simulink model "crossroad_cs"  (R2021a)
settings: Solver=ode5  StartTime=0.0  StopTime=50  FixedStep=1/1000  RelTol=1e-3
PreLoadFcn:
  | mbxruntime.callbacks.PreLoadFcn(bdroot);
PostLoadFcn:
  | mbxruntime.callbacks.PostLoadFcn(bdroot);
InitFcn:
  | mbxruntime.callbacks.InitFcn(bdroot);
StartFcn:
  | mbxruntime.callbacks.StartFcn(bdroot);
StopFcn:
  | mbxruntime.callbacks.StopFcn(bdroot);
model workspace: external: MAT-File .\crossroad_cs_hws.mat (data not in the file)
values from neighbouring files (symbols this model uses):
  c_factor = 43.75    [emplanner_init.m]
  cf = -175016    [emplanner_init.m]
  cr = -130634    [emplanner_init.m]
  KD_PID_distance = 0.0    (= 0)    [emplanner_init.m]
  KD_PID_speed = 0    [emplanner_init.m]
  KI_PID_distance = 0.0    (= 0)    [emplanner_init.m]
  KI_PID_speed = 0    [emplanner_init.m]
  KP_PID_distance = 0.5    [emplanner_init.m]
  KP_PID_speed = 1.8    [emplanner_init.m]
  la = 1.265    [emplanner_init.m]
  lb = 2.947-1.265    (= 1.682)    [emplanner_init.m]
  LQR_K1 = k(:,1)'    [emplanner_init.m]
  LQR_K2 = k(:,2)'    [emplanner_init.m]
  LQR_K3 = k(:,3)'    [emplanner_init.m]
  LQR_K4 = k(:,4)'    [emplanner_init.m]
  m = 2020    [emplanner_init.m]
  my_global_path_x = [0.4409 0.940746626271 1.44028225507 1.93950267328 2.43840536558 2.93698884522 3.43525224935 3.93319509352 4.43081712279 4.92811822143 5.42509835808 5.92175755256 ... (6001 elements, 6001x1)]    [my_global_path.mat]    (also in my_global_path_200.mat = [0.4409 0.940746626271 1.44028225507 1.93950267328 2.4384053)
  my_global_path_y = [58.2244 58.2243999975 58.2243999675 58.2243998683 58.224399668 58.2243993499 58.2243989099 58.2243983526 58.2243976886 58.2243969324 58.2243961011 58.2243952132 ... (6001 elements, 6001x1)]    [my_global_path.mat]    (also in my_global_path_200.mat = [58.2244 58.2243999975 58.2243999675 58.2243998683 58.224399)
  rack_displacement = [-39.14 , -37.2 , -35.29 , -33.43 , -31.6 , -29.81 , -28.06 , -26.34 , -24.66 ,      -23.01 , -21.38 , -19.79 , -18.23 , -16.69 , -15.18 , -13.7 , -12.23 , -10.8 , -9.38 , -7.98 ,     -6.61 , -5.25 , -3.91 , -2.59 , -1.29 , 0 , 1.27 , 2.54 , 3.78 , 5.02 , 6.24 , 7.46 , 8.66 ,      9.86 , 11.05 , 12.24 , 13.41 , 14.59 , 15.76 , 16.92 , 18.09 , 19.25 , 20.42 , 21.59 , 22.76 ,      23.93 , 25.11 , 26 ...(+26 chars)    [emplanner_init.m]
  right_wheel_ground = [-70 ,-67.2 , -64.4 , -61.6 , -58.8 , -56 , -53.2 , -50.4 , -47.6 , -44.8 , -42 ,      -39.2 , -36.4 , -33.6 , -30.8 , -28 , -25.2 , -22.4 , -19.6 , -16.8 , -14 , -11.2 , -8.4 , -5.6 ,      -2.8 , 0 , 2.8 , 5.6 , 8.4 , 11.2 , 14 , 16.8 , 19.6 , 22.4 , 25.2 , 28 , 30.8 , 33.6 , 36.4 ,      39.2 , 42 , 44.8 , 47.6 , 50.4 , 53.2 , 56 , 58.8 , 61.6 , 64.4 , 67.2 , 70 ]    [emplanner_init.m]
  vx_break_point = zeros(1,5000)    [emplanner_init.m]
undefined symbols (not defined in the file or in its folder): aubr, DiscIntNeverNeededParam, tablebr, vubr
libraries: PreScanSimulinkLibrary x11, Solver_SF x1
(part 4 of 8)

== system crossroad_cs/Box_3/Dynamics_Empty/MuxState ==
  note: mode: Dynamics
  note: mode: Positioning
  note: mode: Dynamics
      | VelVEHICLE
      | wrt VEH
  note: AnglesVEHICLE
      | wrtGLOB
  note: For state mode 'Dynamic' positions
      | are not taken into account, as they
      | are computed by integrating velocity.
      | Click annotation for Help.
  x [m] : Inport  SampleTime=TimeStep
  y [m] : Inport  Port=2  SampleTime=TimeStep
  z [m] : Inport  Port=3  SampleTime=TimeStep
  dx [m/s] : Inport  Port=4  SampleTime=TimeStep
  dy [m/s] : Inport  Port=5  SampleTime=TimeStep
  dz [m/s] : Inport  Port=6  SampleTime=TimeStep
  R [rad] : Inport  Port=7  SampleTime=TimeStep
  P [rad] : Inport  Port=8  SampleTime=TimeStep
  Y [rad] : Inport  Port=9  SampleTime=TimeStep
  Constant : Constant  DisableCoverage=on  Value=positioningmode
  Discrete-Time Integrator : DiscreteIntegrator  SampleTime=TimeStep  ICPrevOutput=DiscIntNeverNeededParam  ICPrevScaledInput=DiscIntNeverNeededParam
  Ground : Ground
  Ground1 : Ground
  Mux1 : Mux  Inputs=[3 3]
  Mux2 : Mux  Inputs=3
  Mux3 : Mux  Inputs=3
  Mux4 : Mux  Inputs=3
  Mux5 : Mux  Inputs=[3 3]
  Mux6 : Mux  Inputs=[6 3]
  Switch : Switch  Threshold=0.5
  Transformation_BODY2GLOBAL : PreScanSimulinkLibrary/Simple_Vehicle_Dynamics/Chassis/MuxDynState/Transformation_BODY2GLOBAL  SystemSampleTime=-1  VariantActivationTime=update diagram  Latency=0  AutoFrameSizeCalculation=off
  mux3 : Mux  Inputs=3
  state : Outport
  wires:
  Constant/1 -> Switch/2
  Mux6/1 -> state/1
  Mux4/1 -> Mux1/1
  Mux5/1 -> Switch/3
  Mux1/1 -> Switch/1
  Switch/1 -> Mux6/1  "PosVeh wrt  GLOB"
  P [rad]/1 -> Mux3/2
  R [rad]/1 -> Mux3/1
  dz [m/s]/1 -> Mux2/3
  dy [m/s]/1 -> Mux2/2
  dx [m/s]/1 -> Mux2/1
  z [m]/1 -> Mux4/3
  y [m]/1 -> Mux4/2
  x [m]/1 -> Mux4/1
  Ground1/1 -> mux3/2  "pitch"
  Y [rad]/1 -> mux3/3, Mux3/3  "yaw"
  Mux3/1 -> Mux6/2
  Transformation_BODY2GLOBAL/1 -> Discrete-Time Integrator/1, Mux5/2  "VelVEH wrt  GLOB"
  mux3/1 -> Transformation_BODY2GLOBAL/2
  Ground/1 -> mux3/1  "roll"
  Mux2/1 -> Mux1/2, Transformation_BODY2GLOBAL/1
  Discrete-Time Integrator/1 -> Mux5/1  "PosVEH wrt  GLOB"

== system crossroad_cs/Box_3/Dynamics_Empty/STATE_Box_3 ==
  State : Inport  SampleTime=TimeStep
  Bus Creator : BusCreator  Inputs=15  OutDataTypeStr=Bus: PRESCAN_STATEACTUATORDATA  NonVirtualBus=on
  Constant : Constant  Value=0
  Demux : Demux  Outputs=15
  Mux : Mux  Inputs=3
  Mux1 : Mux  Inputs=3
  Mux2 : Mux  Inputs=3
  iniBODYAngles wrtVEH [rad] : Constant  Value=Roll0  SampleTime=TimeStep
  iniBODYAngles wrtVEH [rad]1 : Constant  Value=Pitch0  SampleTime=TimeStep
  iniVEHAngles wrtGLOB [rad] : Constant  Value=Yaw0  SampleTime=TimeStep
  iniVEHposition wrtGLOB [m] : Constant  Value=x0  SampleTime=TimeStep
  iniVEHposition wrtGLOB [m]1 : Constant  Value=y0  SampleTime=TimeStep
  iniVEHposition wrtGLOB [m]2 : Constant  Value=z0  SampleTime=TimeStep
  state2FullState : PreScanSimulinkLibrary/state2FullState  SystemSampleTime=-1  VariantActivationTime=update diagram  Latency=0  AutoFrameSizeCalculation=off
  StateBus : Outport  OutDataTypeStr=Bus: PRESCAN_STATEACTUATORDATA
  wires:
  Mux2/1 -> state2FullState/4
  iniVEHAngles wrtGLOB [rad]/1 -> Mux2/3
  Mux1/1 -> state2FullState/3
  Constant/1 -> Mux2/1, Mux2/2, Mux1/3
  iniBODYAngles wrtVEH [rad]1/1 -> Mux1/2
  iniBODYAngles wrtVEH [rad]/1 -> Mux1/1
  Mux/1 -> state2FullState/2
  iniVEHposition wrtGLOB [m]2/1 -> Mux/3
  iniVEHposition wrtGLOB [m]/1 -> Mux/1
  iniVEHposition wrtGLOB [m]1/1 -> Mux/2
  Demux/15 -> Bus Creator/15  "AngularVelocityYaw"
  Demux/14 -> Bus Creator/14  "AngularVelocityPitch"
  Demux/13 -> Bus Creator/13  "AngularVelocityRoll"
  Demux/12 -> Bus Creator/12  "OrientationYaw"
  Demux/11 -> Bus Creator/11  "OrientationPitch"
  Demux/10 -> Bus Creator/10  "OrientationRoll"
  Demux/9 -> Bus Creator/9  "AccelerationZ"
  Demux/8 -> Bus Creator/8  "AccelerationY"
  Demux/7 -> Bus Creator/7  "AccelerationX"
  Demux/6 -> Bus Creator/6  "VelocityZ"
  Demux/5 -> Bus Creator/5  "VelocityY"
  Demux/4 -> Bus Creator/4  "VelocityX"
  Demux/3 -> Bus Creator/3  "PositionZ"
  Demux/2 -> Bus Creator/2  "PositionY"
  Demux/1 -> Bus Creator/1  "PositionX"
  state2FullState/1 -> Demux/1
  State/1 -> state2FullState/1
  Bus Creator/1 -> StateBus/1

== system crossroad_cs/Box_3/SELF_Demux/compas converter ==
  rotz [rad] : Inport
  cart2compas : Subsystem
  rad2deg : Gain  Gain=180/pi
  heading [deg] : Outport
  wires:
  rad2deg/1 -> cart2compas/1(Angle [deg])
  rotz [rad]/1 -> rad2deg/1
  cart2compas/1(heading [deg]) -> heading [deg]/1

== system crossroad_cs/Box_4/Dynamics_Empty/MuxState ==
  note: mode: Dynamics
  note: mode: Positioning
  note: mode: Dynamics
      | VelVEHICLE
      | wrt VEH
  note: AnglesVEHICLE
      | wrtGLOB
  note: For state mode 'Dynamic' positions
      | are not taken into account, as they
      | are computed by integrating velocity.
      | Click annotation for Help.
  x [m] : Inport  SampleTime=TimeStep
  y [m] : Inport  Port=2  SampleTime=TimeStep
  z [m] : Inport  Port=3  SampleTime=TimeStep
  dx [m/s] : Inport  Port=4  SampleTime=TimeStep
  dy [m/s] : Inport  Port=5  SampleTime=TimeStep
  dz [m/s] : Inport  Port=6  SampleTime=TimeStep
  R [rad] : Inport  Port=7  SampleTime=TimeStep
  P [rad] : Inport  Port=8  SampleTime=TimeStep
  Y [rad] : Inport  Port=9  SampleTime=TimeStep
  Constant : Constant  DisableCoverage=on  Value=positioningmode
  Discrete-Time Integrator : DiscreteIntegrator  SampleTime=TimeStep  ICPrevOutput=DiscIntNeverNeededParam  ICPrevScaledInput=DiscIntNeverNeededParam
  Ground : Ground
  Ground1 : Ground
  Mux1 : Mux  Inputs=[3 3]
  Mux2 : Mux  Inputs=3
  Mux3 : Mux  Inputs=3
  Mux4 : Mux  Inputs=3
  Mux5 : Mux  Inputs=[3 3]
  Mux6 : Mux  Inputs=[6 3]
  Switch : Switch  Threshold=0.5
  Transformation_BODY2GLOBAL : PreScanSimulinkLibrary/Simple_Vehicle_Dynamics/Chassis/MuxDynState/Transformation_BODY2GLOBAL  SystemSampleTime=-1  VariantActivationTime=update diagram  Latency=0  AutoFrameSizeCalculation=off
  mux3 : Mux  Inputs=3
  state : Outport
  wires:
  Constant/1 -> Switch/2
  Mux6/1 -> state/1
  Mux4/1 -> Mux1/1
  Mux5/1 -> Switch/3
  Mux1/1 -> Switch/1
  Switch/1 -> Mux6/1  "PosVeh wrt  GLOB"
  P [rad]/1 -> Mux3/2
  R [rad]/1 -> Mux3/1
  dz [m/s]/1 -> Mux2/3
  dy [m/s]/1 -> Mux2/2
  dx [m/s]/1 -> Mux2/1
  z [m]/1 -> Mux4/3
  y [m]/1 -> Mux4/2
  x [m]/1 -> Mux4/1
  Ground1/1 -> mux3/2  "pitch"
  Y [rad]/1 -> mux3/3, Mux3/3  "yaw"
  Mux3/1 -> Mux6/2
  Transformation_BODY2GLOBAL/1 -> Discrete-Time Integrator/1, Mux5/2  "VelVEH wrt  GLOB"
  mux3/1 -> Transformation_BODY2GLOBAL/2
  Ground/1 -> mux3/1  "roll"
  Mux2/1 -> Mux1/2, Transformation_BODY2GLOBAL/1
  Discrete-Time Integrator/1 -> Mux5/1  "PosVEH wrt  GLOB"

== system crossroad_cs/Box_4/Dynamics_Empty/STATE_Box_4 ==
  State : Inport  SampleTime=TimeStep
  Bus Creator : BusCreator  Inputs=15  OutDataTypeStr=Bus: PRESCAN_STATEACTUATORDATA  NonVirtualBus=on
  Constant : Constant  Value=0
  Demux : Demux  Outputs=15
  Mux : Mux  Inputs=3
  Mux1 : Mux  Inputs=3
  Mux2 : Mux  Inputs=3
  iniBODYAngles wrtVEH [rad] : Constant  Value=Roll0  SampleTime=TimeStep
  iniBODYAngles wrtVEH [rad]1 : Constant  Value=Pitch0  SampleTime=TimeStep
  iniVEHAngles wrtGLOB [rad] : Constant  Value=Yaw0  SampleTime=TimeStep
  iniVEHposition wrtGLOB [m] : Constant  Value=x0  SampleTime=TimeStep
  iniVEHposition wrtGLOB [m]1 : Constant  Value=y0  SampleTime=TimeStep
  iniVEHposition wrtGLOB [m]2 : Constant  Value=z0  SampleTime=TimeStep
  state2FullState : PreScanSimulinkLibrary/state2FullState  SystemSampleTime=-1  VariantActivationTime=update diagram  Latency=0  AutoFrameSizeCalculation=off
  StateBus : Outport  OutDataTypeStr=Bus: PRESCAN_STATEACTUATORDATA
  wires:
  Mux2/1 -> state2FullState/4
  iniVEHAngles wrtGLOB [rad]/1 -> Mux2/3
  Mux1/1 -> state2FullState/3
  Constant/1 -> Mux2/1, Mux2/2, Mux1/3
  iniBODYAngles wrtVEH [rad]1/1 -> Mux1/2
  iniBODYAngles wrtVEH [rad]/1 -> Mux1/1
  Mux/1 -> state2FullState/2
  iniVEHposition wrtGLOB [m]2/1 -> Mux/3
  iniVEHposition wrtGLOB [m]/1 -> Mux/1
  iniVEHposition wrtGLOB [m]1/1 -> Mux/2
  Demux/15 -> Bus Creator/15  "AngularVelocityYaw"
  Demux/14 -> Bus Creator/14  "AngularVelocityPitch"
  Demux/13 -> Bus Creator/13  "AngularVelocityRoll"
  Demux/12 -> Bus Creator/12  "OrientationYaw"
  Demux/11 -> Bus Creator/11  "OrientationPitch"
  Demux/10 -> Bus Creator/10  "OrientationRoll"
  Demux/9 -> Bus Creator/9  "AccelerationZ"
  Demux/8 -> Bus Creator/8  "AccelerationY"
  Demux/7 -> Bus Creator/7  "AccelerationX"
  Demux/6 -> Bus Creator/6  "VelocityZ"
  Demux/5 -> Bus Creator/5  "VelocityY"
  Demux/4 -> Bus Creator/4  "VelocityX"
  Demux/3 -> Bus Creator/3  "PositionZ"
  Demux/2 -> Bus Creator/2  "PositionY"
  Demux/1 -> Bus Creator/1  "PositionX"
  state2FullState/1 -> Demux/1
  State/1 -> state2FullState/1
  Bus Creator/1 -> StateBus/1

== system crossroad_cs/Box_4/SELF_Demux/compas converter ==
  rotz [rad] : Inport
  cart2compas : Subsystem
  rad2deg : Gain  Gain=180/pi
  heading [deg] : Outport
  wires:
  rad2deg/1 -> cart2compas/1(Angle [deg])
  rotz [rad]/1 -> rad2deg/1
  cart2compas/1(heading [deg]) -> heading [deg]/1

== system crossroad_cs/Audi_A8_Sedan_1/Dynamics_UserSpecified/CarSim2PreScanSTATE/Transformation_SprungMassCarSim2PreScan ==
  In1 : Inport
  Demux : Demux  Outputs=3
  Ini z-position VEHICLE wrt GLOBAL axis system [m] : Constant  Value=z0
  Mux : Mux  Inputs=3
  Sum1 : Sum  Inputs=+-
  Out1 : Outport
  wires:
  Mux/1 -> Out1/1
  Ini z-position VEHICLE wrt GLOBAL axis system [m]/1 -> Sum1/2
  Demux/1 -> Mux/1
  Sum1/1 -> Mux/3
  Demux/3 -> Sum1/1
  Demux/2 -> Mux/2
  In1/1 -> Demux/1

== system crossroad_cs/Audi_A8_Sedan_1/SELF_Demux/compas converter/cart2compas ==
  Angle [deg] : Inport
  Constant : Constant  Value=90
  Constant1 : Constant  Value=360
  Gain : Gain  Gain=1/360
  Gain1 : Gain  Gain=360
  Gain2 : Gain  Gain=-1
  Rounding Function : Rounding
  Sum : Sum  Inputs=|-+
  Sum1 : Sum  Inputs=-+|
  Sum2 : Sum  Inputs=++|
  heading [deg] : Outport
  wires:
  Gain/1 -> Rounding Function/1
  Rounding Function/1 -> Gain1/1
  Gain1/1 -> Sum/1
  Angle [deg]/1 -> Sum1/2
  Sum/1 -> Gain2/1
  Sum1/1 -> Gain/1, Sum/2
  Constant/1 -> Sum1/1
  Gain2/1 -> Sum2/2
  Constant1/1 -> Sum2/1
  Sum2/1 -> heading [deg]/1

== system crossroad_cs/Audi_A8_Sedan_1/control module1/control main/chassic steering system ==
  LQR_final_angle : Inport
  Constant : Constant  Value=la
  Constant1 : Constant  Value=lb
  Constant17 : Constant  Value=c_factor
  Divide : Product  Inputs=*/
  Gain3 : Gain  Gain=180/pi
  Gain4 : Gain  Gain=360
  MATLAB Function : MATLAB Function  TreatAsAtomicUnit=on
  Saturation : Saturate  UpperLimit=70  LowerLimit=-70
  Saturation1 : Saturate  UpperLimit=1.2217  LowerLimit=-1.2217
  transfer right wheel angle to rack displancement : Lookup_n-D  NumberOfTableDimensions=1  BreakpointsForDimension1=right_wheel_ground  Table=rack_displacement  InternalRulePriority=Speed  RndMeth=Simplest  InputSameDT=on
  lat_steer_sw[deg] : Outport
  wires:
  transfer right wheel angle to rack displancement/1 -> Divide/1
  Constant17/1 -> Divide/2
  Gain4/1 -> lat_steer_sw[deg]/1
  Divide/1 -> Gain4/1
  Saturation/1 -> transfer right wheel angle to rack displancement/1
  Constant/1 -> MATLAB Function/2(la)
  Gain3/1 -> Saturation/1
  Constant1/1 -> MATLAB Function/3(lb)
  LQR_final_angle/1 -> Saturation1/1
  Saturation1/1 -> MATLAB Function/1(u)
  MATLAB Function/1(right_steer) -> Gain3/1

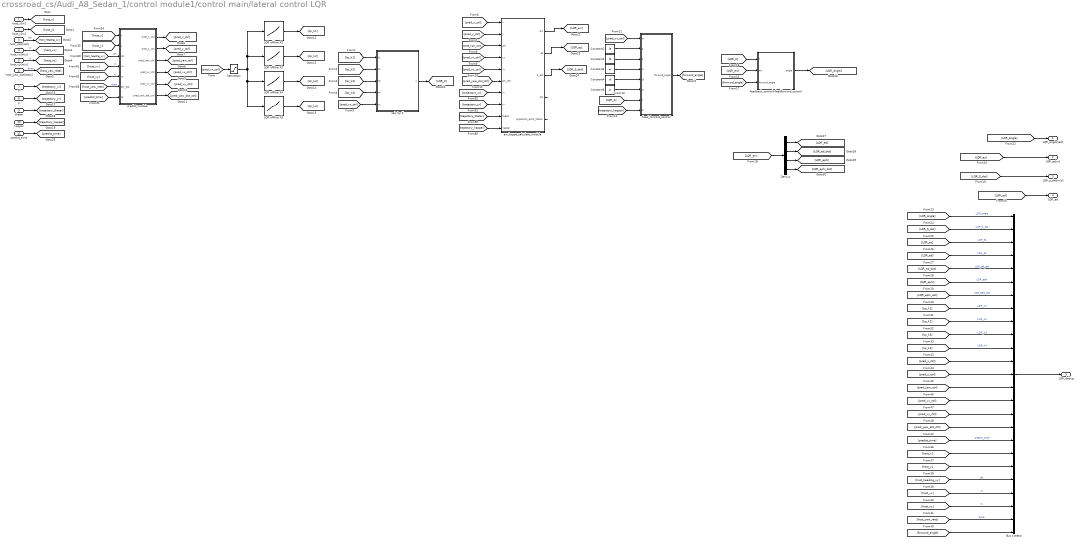
== system crossroad_cs/Audi_A8_Sedan_1/control module1/control main/lateral control LQR ==
  host_x[m] : Inport
  host_y[m] : Inport  Port=2
  host_yaw[rad] : Inport  Port=3
  host_vx[m/s] : Inport  Port=4
  host_vy[m/s] : Inport  Port=5
  host_yaw_dot[rad/s] : Inport  Port=6
  xr : Inport  Port=7
  yr : Inport  Port=8
  thetar : Inport  Port=9
  kappar : Inport  Port=10
  predict_time : Inport  Port=11
  Bus Creator : BusCreator  Inputs=25
  Constant1 : Constant  Value=la
  Constant2 : Constant  Value=lb
  Constant3 : Constant  Value=m
  Constant4 : Constant  Value=cf
  Constant5 : Constant  Value=cr
  Demux : Demux
  LQR offline K1 : Lookup_n-D  NumberOfTableDimensions=1  BreakpointsForDimension1=vx_break_point  Table=LQR_K1  InternalRulePriority=Speed  RndMeth=Simplest  InputSameDT=on
  LQR offline K2 : Lookup_n-D  NumberOfTableDimensions=1  BreakpointsForDimension1=vx_break_point  Table=LQR_K2  InternalRulePriority=Speed  RndMeth=Simplest  InputSameDT=on
  LQR offline K3 : Lookup_n-D  NumberOfTableDimensions=1  BreakpointsForDimension1=vx_break_point  Table=LQR_K3  InternalRulePriority=Speed  RndMeth=Simplest  InputSameDT=on
  LQR offline K4 : Lookup_n-D  NumberOfTableDimensions=1  BreakpointsForDimension1=vx_break_point  Table=LQR_K4  InternalRulePriority=Speed  RndMeth=Simplest  InputSameDT=on
  Saturation : Saturate  UpperLimit=50  LowerLimit=0
  calc lqr K : MATLAB Function  TreatAsAtomicUnit=on
  err_kappa_calculate_module : MATLAB Function  TreatAsAtomicUnit=on
  feed_forword_control : MATLAB Function  TreatAsAtomicUnit=on
  feedback_control+feedforword_control : MATLAB Function  TreatAsAtomicUnit=on
  predict_module : MATLAB Function  TreatAsAtomicUnit=on
  LQR_angle[rad] : Outport  VectorParamsAs1DForOutWhenUnconnected=off
  LQR_es[m] : Outport  Port=2  VectorParamsAs1DForOutWhenUnconnected=off
  LQR_s_dot[m/s] : Outport  Port=3  VectorParamsAs1DForOutWhenUnconnected=off
  LQR_ed : Outport  Port=4  VectorParamsAs1DForOutWhenUnconnected=off
  LQR_debug : Outport  Port=5  VectorParamsAs1DForOutWhenUnconnected=off
  wires:
  [host_vy] -> predict_module/5(vy)  "vy"
  [host_x] -> predict_module/1(x)
  [host_yaw_rate] -> predict_module/6(phi_dot)  "dyaw"
  [host_vx] -> predict_module/4(vx)  "vx"
  [host_y] -> predict_module/2(y)
  [host_heading_xy] -> predict_module/3(phi)  "phi"
  [predict_time] -> predict_module/7(ts)
  host_x[m]/1 -> [host_x]
  host_y[m]/1 -> [host_y]
  host_yaw[rad]/1 -> [host_heading_xy]  "phi"
  host_vx[m/s]/1 -> [host_vx]  "vx"
  host_vy[m/s]/1 -> [host_vy]  "vy"
  host_yaw_dot[rad/s]/1 -> [host_yaw_rate]  "dyaw"
  predict_module/1(pred_x_ctrl) -> [pred_x_ctrl]
  predict_module/2(pred_y_ctrl) -> [pred_y_ctrl]
  predict_module/3(pred_yaw_ctrl) -> [pred_yaw_ctrl]
  predict_module/4(pred_vx_ctrl) -> [pred_vx_ctrl]
  predict_module/5(pred_vy_ctrl) -> [pred_vy_ctrl]
  predict_module/6(pred_yaw_dot_ctrl) -> [pred_yaw_dot_ctrl]
  [pred_vx_ctrl] -> Saturation/1
  LQR offline K1/1 -> [lqr_k1]
  LQR offline K2/1 -> [lqr_k2]
  LQR offline K4/1 -> [lqr_k3]
  LQR offline K3/1 -> [lqr_k4]
  [pred_vx_ctrl] -> calc lqr K/5(vx)
  [lqr_k4] -> calc lqr K/4(k4)
  [lqr_k3] -> calc lqr K/3(k3)
  [lqr_k2] -> calc lqr K/2(k2)
  [lqr_k1] -> calc lqr K/1(k1)
  [pred_x_ctrl] -> err_kappa_calculate_module/1(x)
  [pred_y_ctrl] -> err_kappa_calculate_module/2(y)
  [pred_yaw_ctrl] -> err_kappa_calculate_module/3("phi ")
  [pred_vx_ctrl] -> err_kappa_calculate_module/4(vx)
  [pred_vy_ctrl] -> err_kappa_calculate_module/5(vy)
  [pred_yaw_dot_ctrl] -> err_kappa_calculate_module/6(phi_dot)
  xr/1 -> [trajectory_xr]
  yr/1 -> [trajectory_yr]
  thetar/1 -> [trajectory_thetar]
  kappar/1 -> [trajectory_kappar]
  [trajectory_xr] -> err_kappa_calculate_module/7(xr)
  [trajectory_yr] -> err_kappa_calculate_module/8(yr)
  [trajectory_kappar] -> err_kappa_calculate_module/10(kappar)
  [trajectory_thetar] -> err_kappa_calculate_module/9(thetar)
  [pred_vx_ctrl] -> feed_forword_control/1(vx)
  Constant1/1 -> feed_forword_control/2(a)
  Constant2/1 -> feed_forword_control/3(b)
  Constant3/1 -> feed_forword_control/4(m)
  Constant4/1 -> feed_forword_control/5(cf)
  Constant5/1 -> feed_forword_control/6(cr)
  calc lqr K/1(k) -> [LQR_K]
  [LQR_K] -> feed_forword_control/7(k)
  [trajectory_kappar] -> feed_forword_control/8(kr)
  feed_forword_control/1(forword_angle) -> [forword_angle]
  err_kappa_calculate_module/1(err) -> [LQR_err]
  [LQR_err] -> feedback_control+feedforword_control/2(err)
  [LQR_K] -> feedback_control+feedforword_control/1(k)
  [forword_angle] -> feedback_control+feedforword_control/3(forword_angle)
  [LQR_err] -> Demux/1
  err_kappa_calculate_module/2(es) -> [LQR_es]
  err_kappa_calculate_module/3(s_dot) -> [LQR_S_dot]
  [LQR_S_dot] -> LQR_s_dot[m/s]/1
  [LQR_es] -> LQR_es[m]/1
  Saturation/1 -> LQR offline K3/1, LQR offline K4/1, LQR offline K2/1, LQR offline K1/1
  predict_time/1 -> [predict_time]
  Bus Creator/1 -> LQR_debug/1
  feedback_control+feedforword_control/1(angle) -> [LQR_Angle]
  [LQR_Angle] -> LQR_angle[rad]/1
  [LQR_Angle] -> Bus Creator/1  "LQR_angle"
  [LQR_S_dot] -> Bus Creator/2  "LQR_s_dot"
  [LQR_es] -> Bus Creator/3  "LQR_es"
  Demux/1 -> [LQR_ed]
  Demux/2 -> [LQR_ed_dot]
  Demux/3 -> [LQR_ephi]
  Demux/4 -> [LQR_ephi_dot]
  [LQR_ed] -> Bus Creator/4  "LQR_ed"
  [LQR_ed_dot] -> Bus Creator/5  "LQR_ed_dot"
  [LQR_ephi] -> Bus Creator/6  "LQR_ephi"
  [LQR_ephi_dot] -> Bus Creator/7  "LQR_ephi_dot"
  [lqr_k1] -> Bus Creator/8  "LQR_K1"
  [lqr_k2] -> Bus Creator/9  "LQR_K2"
  [lqr_k3] -> Bus Creator/10  "LQR_K3"
  [lqr_k4] -> Bus Creator/11  "LQR_K4"
  [pred_x_ctrl] -> Bus Creator/12
  [pred_y_ctrl] -> Bus Creator/13
  [pred_yaw_ctrl] -> Bus Creator/14
  [pred_vx_ctrl] -> Bus Creator/15
  [pred_vy_ctrl] -> Bus Creator/16
  [pred_yaw_dot_ctrl] -> Bus Creator/17
  [predict_time] -> Bus Creator/18  "predict_time"
  [host_x] -> Bus Creator/19
  [host_y] -> Bus Creator/20
  [host_heading_xy] -> Bus Creator/21  "phi"
  [host_vx] -> Bus Creator/22  "vx"
  [host_vy] -> Bus Creator/23  "vy"
  [host_yaw_rate] -> Bus Creator/24  "dyaw"
  [forword_angle] -> Bus Creator/25
  [LQR_ed] -> LQR_ed/1
  err_kappa_calculate_module/4(phi) -> ?
  err_kappa_calculate_module/5(projection_point_thetar) -> ?

== system crossroad_cs/Audi_A8_Sedan_1/control module1/control main/longitudinal control double PID ==
  s_err[m] : Inport
  speed_desire[m/s] : Inport  Port=2
  accelerate desire[m/s^2] : Inport  Port=3
  host_speed[m/s] : Inport  Port=4
  host_s_dot[m/s] : Inport  Port=5
  KP_PID_distance : Inport  Port=6
  KI_PID_distance : Inport  Port=7
  KD_PID_distance : Inport  Port=8
  KP_PID_speed : Inport  Port=9
  KI_PID_speed : Inport  Port=10
  KD_PID_speed : Inport  Port=11
  2-D Lookup Table : Lookup_n-D  BreakpointsForDimension1=vubr  BreakpointsForDimension2=aubr  Table=tablebr  InternalRulePriority=Speed  RndMeth=Simplest  InputSameDT=on
      settings: InputPortMap=u0,u1
  Add : Sum  Inputs=++-
  Add1 : Sum
  Bus Creator : BusCreator  Inputs=9
  Discrete Filter : DiscreteFilter
  MATLAB Function1 : MATLAB Function  TreatAsAtomicUnit=on
  Saturation : Saturate  UpperLimit=45  LowerLimit=-45
  Saturation1 : Saturate  UpperLimit=5  LowerLimit=-8
  discrete pid : Subsystem
  discrete pid1 : Subsystem
  throttle : Outport
  brake : Outport  Port=2
  longitudinal_debug : Outport  Port=3
  wires:
  2-D Lookup Table/1 -> MATLAB Function1/1(u)
  s_err[m]/1 -> [s_err]
  speed_desire[m/s]/1 -> [speed_desire]
  accelerate desire[m/s^2]/1 -> [accelerate_desire]
  KP_PID_distance/1 -> [KP_PID_distance]
  KI_PID_distance/1 -> [KI_PID_distance]
  KD_PID_distance/1 -> [KD_PID_distance]
  KP_PID_speed/1 -> [KP_PID_speed]
  KI_PID_speed/1 -> [KI_PID_speed]
  KD_PID_speed/1 -> [KD_PID_speed]
  [s_err] -> Discrete Filter/1
  host_speed[m/s]/1 -> [host_speed]
  [speed_desire] -> Add/2
  Add/1 -> Saturation/1
  Saturation/1 -> discrete pid1/1(err)
  discrete pid1/1(pid_out) -> Add1/1
  [accelerate_desire] -> Add1/2
  Add1/1 -> Saturation1/1
  Saturation1/1 -> 2-D Lookup Table/2
  host_s_dot[m/s]/1 -> [host_s_dot]
  [host_s_dot] -> Add/3
  [host_speed] -> 2-D Lookup Table/1
  MATLAB Function1/1(throttle) -> throttle/1
  MATLAB Function1/2(brake) -> brake/1
  [KP_PID_distance] -> Bus Creator/1  "KP_PID_distance"
  [KI_PID_distance] -> Bus Creator/2  "KI_PID_distance"
  [KD_PID_distance] -> Bus Creator/3  "KD_PID_distance"
  [KP_PID_speed] -> Bus Creator/4  "KP_PID_speed"
  [KI_PID_speed] -> Bus Creator/5  "KI_PID_speed"
  [KD_PID_speed] -> Bus Creator/6  "KD_PID_speed"
  [host_speed] -> Bus Creator/7  "host_speed"
  [s_err] -> Bus Creator/8  "s_err"
  [host_s_dot] -> Bus Creator/9  "host_s_dot"
  Bus Creator/1 -> longitudinal_debug/1
  Discrete Filter/1 -> discrete pid/1(err)
  [KP_PID_distance] -> discrete pid/2(kp)
  [KI_PID_distance] -> discrete pid/3(ki)
  [KD_PID_distance] -> discrete pid/4(kd)
  [KP_PID_speed] -> discrete pid1/2(kp)
  [KI_PID_speed] -> discrete pid1/3(ki)
  [KD_PID_speed] -> discrete pid1/4(kd)
  discrete pid/1(pid_out) -> Add/1

== system crossroad_cs/Audi_A8_Sedan_1/control module1/control main/understeer compensate ==
  LQR_angle : Inport
  lateral err : Inport  Port=2
  Add : Sum  Inputs=+-
  Gain : Gain  Gain=0.01
  Manual Switch : ManualSwitch
  LQR_final_angle : Outport
  wires:
  lateral err/1 -> Gain/1
  Add/1 -> Manual Switch/2
  Manual Switch/1 -> LQR_final_angle/1
  LQR_angle/1 -> Add/1, Manual Switch/1
  Gain/1 -> Add/2

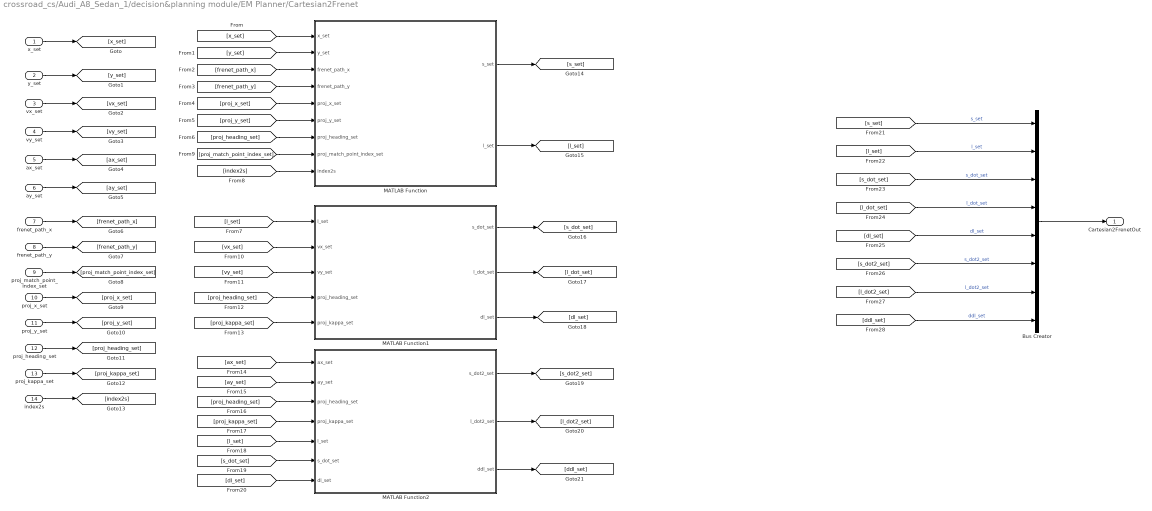
== system crossroad_cs/Audi_A8_Sedan_1/decision&planning module/EM Planner/Cartesian2Frenet ==
  x_set : Inport
  y_set : Inport  Port=2
  vx_set : Inport  Port=3
  vy_set : Inport  Port=4
  ax_set : Inport  Port=5
  ay_set : Inport  Port=6
  frenet_path_x : Inport  Port=7
  frenet_path_y : Inport  Port=8
  proj_match_point_index_set : Inport  Port=9
  proj_x_set : Inport  Port=10
  proj_y_set : Inport  Port=11
  proj_heading_set : Inport  Port=12
  proj_kappa_set : Inport  Port=13
  index2s : Inport  Port=14
  Bus Creator : BusCreator  Inputs=8
  MATLAB Function : MATLAB Function  TreatAsAtomicUnit=on
  MATLAB Function1 : MATLAB Function  TreatAsAtomicUnit=on
  MATLAB Function2 : MATLAB Function  TreatAsAtomicUnit=on
  Cartesian2FrenetOut : Outport
  wires:
  x_set/1 -> [x_set]
  y_set/1 -> [y_set]
  vx_set/1 -> [vx_set]
  vy_set/1 -> [vy_set]
  ax_set/1 -> [ax_set]
  ay_set/1 -> [ay_set]
  frenet_path_x/1 -> [frenet_path_x]
  frenet_path_y/1 -> [frenet_path_y]
  proj_match_point_index_set/1 -> [proj_match_point_index_set]
  proj_x_set/1 -> [proj_x_set]
  proj_y_set/1 -> [proj_y_set]
  proj_heading_set/1 -> [proj_heading_set]
  proj_kappa_set/1 -> [proj_kappa_set]
  index2s/1 -> [index2s]
  [x_set] -> MATLAB Function/1(x_set)
  [y_set] -> MATLAB Function/2(y_set)
  [frenet_path_x] -> MATLAB Function/3(frenet_path_x)
  [frenet_path_y] -> MATLAB Function/4(frenet_path_y)
  [proj_x_set] -> MATLAB Function/5(proj_x_set)
  [proj_match_point_index_set] -> MATLAB Function/8(proj_match_point_index_set)
  [proj_y_set] -> MATLAB Function/6(proj_y_set)
  [proj_heading_set] -> MATLAB Function/7(proj_heading_set)
  [index2s] -> MATLAB Function/9(index2s)
  MATLAB Function/1(s_set) -> [s_set]
  MATLAB Function/2(l_set) -> [l_set]
  [l_set] -> MATLAB Function1/1(l_set)
  [vx_set] -> MATLAB Function1/2(vx_set)
  [vy_set] -> MATLAB Function1/3(vy_set)
  [proj_heading_set] -> MATLAB Function1/4(proj_heading_set)
  [proj_kappa_set] -> MATLAB Function1/5(proj_kappa_set)
  [ax_set] -> MATLAB Function2/1(ax_set)
  [ay_set] -> MATLAB Function2/2(ay_set)
  [proj_heading_set] -> MATLAB Function2/3(proj_heading_set)
  [proj_kappa_set] -> MATLAB Function2/4(proj_kappa_set)
  [l_set] -> MATLAB Function2/5(l_set)
  MATLAB Function1/1(s_dot_set) -> [s_dot_set]
  MATLAB Function1/2(l_dot_set) -> [l_dot_set]
  MATLAB Function1/3(dl_set) -> [dl_set]
  [s_dot_set] -> MATLAB Function2/6(s_dot_set)
  [dl_set] -> MATLAB Function2/7(dl_set)
  MATLAB Function2/1(s_dot2_set) -> [s_dot2_set]
  MATLAB Function2/2(l_dot2_set) -> [l_dot2_set]
  MATLAB Function2/3(ddl_set) -> [ddl_set]
  [s_set] -> Bus Creator/1  "s_set"
  [l_set] -> Bus Creator/2  "l_set"
  [s_dot_set] -> Bus Creator/3  "s_dot_set"
  [l_dot_set] -> Bus Creator/4  "l_dot_set"
  [dl_set] -> Bus Creator/5  "dl_set"
  [s_dot2_set] -> Bus Creator/6  "s_dot2_set"
  [l_dot2_set] -> Bus Creator/7  "l_dot2_set"
  [ddl_set] -> Bus Creator/8  "ddl_set"
  Bus Creator/1 -> Cartesian2FrenetOut/1

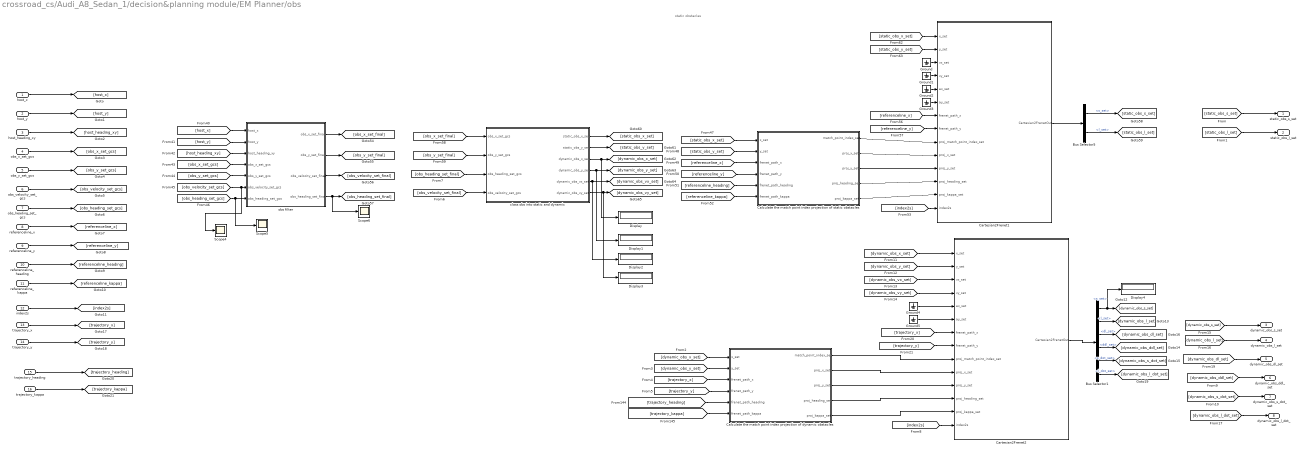
== system crossroad_cs/Audi_A8_Sedan_1/decision&planning module/EM Planner/obs ==
  note: static obstacles
  host_x : Inport
  host_y : Inport  Port=2
  host_heading_xy : Inport  Port=3
  obs_x_set_gcs : Inport  Port=4
  obs_y_set_gcs : Inport  Port=5
  obs_velocity_set_gcs : Inport  Port=6
  obs_heading_set_gcs : Inport  Port=7
  referenceline_x : Inport  Port=8
  referenceline_y : Inport  Port=9
  referenceline_heading : Inport  Port=10
  referenceline_kappa : Inport  Port=11
  index2s : Inport  Port=12
  trajectory_x : Inport  Port=13
  trajectory_y : Inport  Port=14
  trajectory_heading : Inport  Port=15
  trajectory_kappa : Inport  Port=16
  Bus Selector1 : BusSelector  OutputSignals=s_set,l_set,dl_set,ddl_set,s_dot_set,l_dot_set
  Bus Selector5 : BusSelector  OutputSignals=s_set,l_set
  Calculate the match point index projection of dynamic obstacles : MATLAB Function  TreatAsAtomicUnit=on
  Calculate the match point index projection of static obstacles : MATLAB Function  TreatAsAtomicUnit=on
  Cartesian2Frenet1 : Subsystem
  Cartesian2Frenet2 : Subsystem
  Display{,1..4} (5 alike) : Display
  Ground{,1..5} (6 alike) : Ground
  Scope4 : Scope
  Scope5 : Scope
  Scope6 : Scope
  class obs into static and dynamic : MATLAB Function  TreatAsAtomicUnit=on
  obs filter : MATLAB Function  TreatAsAtomicUnit=on
  static_obs_s_set : Outport
  static_obs_l_set : Outport  Port=2
  dynamic_obs_s_set : Outport  Port=3
  dynamic_obs_l_set : Outport  Port=4
  dynamic_obs_dl_set : Outport  Port=5
  dynamic_obs_ddl_set : Outport  Port=6
  dynamic_obs_s_dot_set : Outport  Port=7
  dynamic_obs_l_dot_set : Outport  Port=8
  wires:
  Ground3/1 -> Cartesian2Frenet1/6(ay_set)
  [obs_x_set_gcs] -> obs filter/4(obs_x_set_gcs)
  [index2s] -> Cartesian2Frenet1/14(index2s)
  [referenceline_y] -> Cartesian2Frenet1/8(frenet_path_y)
  Calculate the match point index projection of static obstacles/5(proj_kappa_set) -> Cartesian2Frenet1/13(proj_kappa_set)
  Calculate the match point index projection of static obstacles/4(proj_heading_set) -> Cartesian2Frenet1/12(proj_heading_set)
  [referenceline_x] -> Calculate the match point index projection of static obstacles/3(frenet_path_x)
  Ground2/1 -> Cartesian2Frenet1/5(ax_set)
  obs filter/1(obs_x_set_final) -> [obs_x_set_final]
  obs filter/4(obs_heading_set_final) -> Scope6/1, [obs_heading_set_final]
  [host_heading_xy] -> obs filter/3(host_heading_xy)
  class obs into static and dynamic/5(dynamic_obs_vx_set) -> Display2/1, [dynamic_obs_vx_set]
  [obs_y_set_final] -> class obs into static and dynamic/2(obs_y_set_gcs)
  class obs into static and dynamic/6(dynamic_obs_vy_set) -> Display3/1, [dynamic_obs_vy_set]
  [referenceline_y] -> Calculate the match point index projection of static obstacles/4(frenet_path_y)
  obs filter/3(obs_velocity_set_final) -> [obs_velocity_set_final]
  class obs into static and dynamic/1(static_obs_x_set) -> [static_obs_x_set]
  [obs_heading_set_gcs] -> Scope5/1, obs filter/7(obs_heading_set_gcs)
  [referenceline_kappa] -> Calculate the match point index projection of static obstacles/6(frenet_path_kappa)
  [static_obs_x_set] -> Cartesian2Frenet1/1(x_set)
  [static_obs_y_set] -> Calculate the match point index projection of static obstacles/2(y_set)
  [referenceline_x] -> Cartesian2Frenet1/7(frenet_path_x)
  Ground1/1 -> Cartesian2Frenet1/4(vy_set)
  [obs_x_set_final] -> class obs into static and dynamic/1(obs_x_set_gcs)
  [obs_velocity_set_gcs] -> Scope4/1, obs filter/6(obs_velocity_set_gcs)
  [host_y] -> obs filter/2(host_y)
  Bus Selector5/2 -> [static_obs_l_set]  "<l_set>"
  [referenceline_heading] -> Calculate the match point index projection of static obstacles/5(frenet_path_heading)
  obs filter/2(obs_y_set_final) -> [obs_y_set_final]
  Bus Selector5/1 -> [static_obs_s_set]  "<s_set>"
  class obs into static and dynamic/3(dynamic_obs_x_set) -> Display/1, [dynamic_obs_x_set]
  Calculate the match point index projection of static obstacles/2(proj_x_set) -> Cartesian2Frenet1/10(proj_x_set)
  Ground/1 -> Cartesian2Frenet1/3(vx_set)
  Calculate the match point index projection of static obstacles/3(proj_y_set) -> Cartesian2Frenet1/11(proj_y_set)
  class obs into static and dynamic/4(dynamic_obs_y_set) -> Display1/1, [dynamic_obs_y_set]
  Calculate the match point index projection of static obstacles/1(match_point_index_set) -> Cartesian2Frenet1/9(proj_match_point_index_set)
  [host_x] -> obs filter/1(host_x)
  [obs_y_set_gcs] -> obs filter/5(obs_y_set_gcs)
  Cartesian2Frenet1/1(Cartesian2FrenetOut) -> Bus Selector5/1
  [static_obs_x_set] -> Calculate the match point index projection of static obstacles/1(x_set)
  class obs into static and dynamic/2(static_obs_y_set) -> [static_obs_y_set]
  [static_obs_y_set] -> Cartesian2Frenet1/2(y_set)
  host_x/1 -> [host_x]
  host_y/1 -> [host_y]
  host_heading_xy/1 -> [host_heading_xy]
  obs_x_set_gcs/1 -> [obs_x_set_gcs]
  obs_y_set_gcs/1 -> [obs_y_set_gcs]
  obs_velocity_set_gcs/1 -> [obs_velocity_set_gcs]
  obs_heading_set_gcs/1 -> [obs_heading_set_gcs]
  referenceline_x/1 -> [referenceline_x]
  referenceline_y/1 -> [referenceline_y]
  referenceline_heading/1 -> [referenceline_heading]
  referenceline_kappa/1 -> [referenceline_kappa]
  index2s/1 -> [index2s]
  [static_obs_s_set] -> static_obs_s_set/1
  [static_obs_l_set] -> static_obs_l_set/1
  [dynamic_obs_x_set] -> Calculate the match point index projection of dynamic obstacles/1(x_set)
  [dynamic_obs_y_set] -> Calculate the match point index projection of dynamic obstacles/2(y_set)
  Calculate the match point index projection of dynamic obstacles/1(match_point_index_set) -> Cartesian2Frenet2/9(proj_match_point_index_set)
  Calculate the match point index projection of dynamic obstacles/2(proj_x_set) -> Cartesian2Frenet2/10(proj_x_set)
  Calculate the match point index projection of dynamic obstacles/3(proj_y_set) -> Cartesian2Frenet2/11(proj_y_set)
  Calculate the match point index projection of dynamic obstacles/4(proj_heading_set) -> Cartesian2Frenet2/12(proj_heading_set)
  Calculate the match point index projection of dynamic obstacles/5(proj_kappa_set) -> Cartesian2Frenet2/13(proj_kappa_set)
  [index2s] -> Cartesian2Frenet2/14(index2s)
  [dynamic_obs_x_set] -> Cartesian2Frenet2/1(x_set)
  [dynamic_obs_y_set] -> Cartesian2Frenet2/2(y_set)
  [dynamic_obs_vx_set] -> Cartesian2Frenet2/3(vx_set)
  [dynamic_obs_vy_set] -> Cartesian2Frenet2/4(vy_set)
  Ground4/1 -> Cartesian2Frenet2/5(ax_set)
  Ground5/1 -> Cartesian2Frenet2/6(ay_set)
  Cartesian2Frenet2/1(Cartesian2FrenetOut) -> Bus Selector1/1
  Bus Selector1/1 -> Display4/1, [dynamic_obs_s_set]  "<s_set>"
  Bus Selector1/2 -> [dynamic_obs_l_set]  "<l_set>"
  Bus Selector1/3 -> [dynamic_obs_dl_set]  "<dl_set>"
  [dynamic_obs_s_set] -> dynamic_obs_s_set/1
  [dynamic_obs_l_set] -> dynamic_obs_l_set/1
  [dynamic_obs_dl_set] -> dynamic_obs_dl_set/1
  trajectory_x/1 -> [trajectory_x]
  trajectory_y/1 -> [trajectory_y]
  Bus Selector1/4 -> [dynamic_obs_ddl_set]  "<ddl_set>"
  [dynamic_obs_ddl_set] -> dynamic_obs_ddl_set/1
  Bus Selector1/5 -> [dynamic_obs_s_dot_set]  "<s_dot_set>"
  Bus Selector1/6 -> [dynamic_obs_l_dot_set]  "<l_dot_set>"
  [dynamic_obs_s_dot_set] -> dynamic_obs_s_dot_set/1
  [dynamic_obs_l_dot_set] -> dynamic_obs_l_dot_set/1
  trajectory_heading/1 -> [trajectory_heading]
  trajectory_kappa/1 -> [trajectory_kappa]
  [trajectory_x] -> Calculate the match point index projection of dynamic obstacles/3(frenet_path_x)
  [trajectory_y] -> Calculate the match point index projection of dynamic obstacles/4(frenet_path_y)
  [trajectory_heading] -> Calculate the match point index projection of dynamic obstacles/5(frenet_path_heading)
  [trajectory_kappa] -> Calculate the match point index projection of dynamic obstacles/6(frenet_path_kappa)
  [trajectory_x] -> Cartesian2Frenet2/7(frenet_path_x)
  [trajectory_y] -> Cartesian2Frenet2/8(frenet_path_y)
  [obs_velocity_set_final] -> class obs into static and dynamic/4(obs_velocity_set_gcs)
  [obs_heading_set_final] -> class obs into static and dynamic/3(obs_heading_set_gcs)

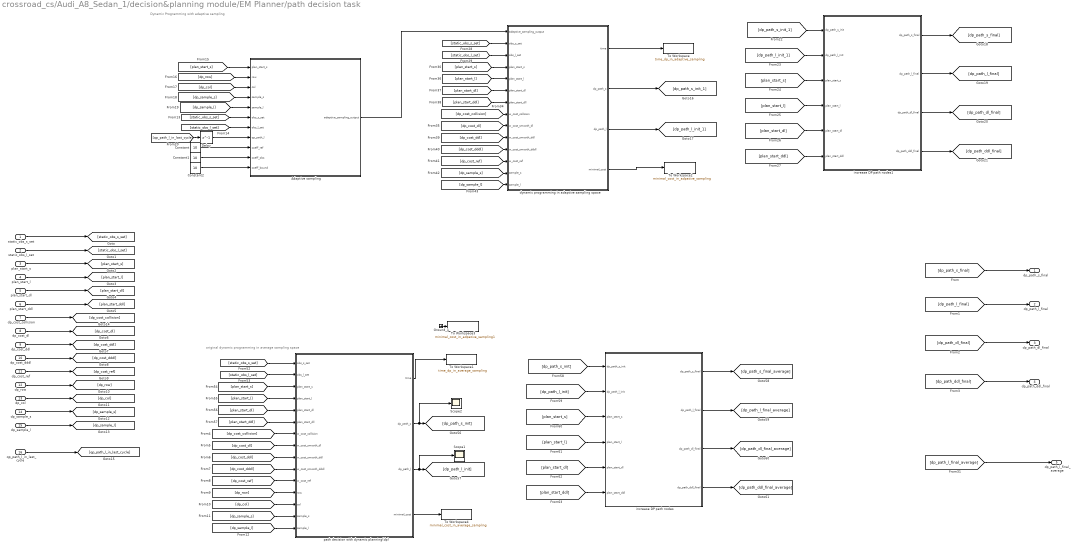
== system crossroad_cs/Audi_A8_Sedan_1/decision&planning module/EM Planner/path decision task ==
  note: Dynamic Programming with adaptive sampling
  note: original dynamic programming in average sampling space
  static_obs_s_set : Inport
  static_obs_l_set : Inport  Port=2
  plan_start_s : Inport  Port=3
  plan_start_l : Inport  Port=4
  plan_start_dl : Inport  Port=5
  plan_start_ddl : Inport  Port=6
  dp_cost_collision : Inport  Port=7
  dp_cost_dl : Inport  Port=8
  dp_cost_ddl : Inport  Port=9
  dp_cost_dddl : Inport  Port=10
  dp_cost_ref : Inport  Port=11
  dp_row : Inport  Port=12
  dp_col : Inport  Port=13
  dp_sample_s : Inport  Port=14
  dp_sample_l : Inport  Port=15
  qp_path_l_in_last_cycle : Inport  Port=16
  Adaptive sampling : MATLAB Function  TreatAsAtomicUnit=on
  Constant : Constant  Value=10
  Constant1 : Constant  Value=10
  Constant2 : Constant  Value=10
  Delay : Delay  DelayLength=1  InitialCondition=[-2 -2 -2 -2 -2 -2 -2 -2 -2 -2 -2 -2 -2 -2 -2 -2 -2 -2 -2 -2 -2 -2 -2 -2 -2 -2 -2 -2 -2 -2 -2 -2 -2 -2 -2 -2 -2 -2 -2 -2 -2 -2 -2 -2 -2 -2 -2 -2 -2 -2 -2 -2 -2 -2 -2 -2 -2 -2 -2 -2]
  Ground_1 : Ground
  Scope1 : Scope
  Scope2 : Scope
  To Workspace : ToWorkspace  VariableName=time_dp_in_adaptive_sampling  SaveFormat=Timeseries  SampleTime=-1
  To Workspace1 : ToWorkspace  VariableName=time_dp_in_average_sampling  SaveFormat=Timeseries  SampleTime=-1
  To Workspace2 : ToWorkspace  VariableName=minimal_cost_in_adpative_sampling  SaveFormat=Timeseries  SampleTime=-1
  To Workspace3 : ToWorkspace  VariableName=minimal_cost_in_adpative_sampling1  SaveFormat=Timeseries  SampleTime=-1
  To Workspace4 : ToWorkspace  VariableName=minimal_cost_in_average_sampling  SaveFormat=Timeseries  SampleTime=-1
  dynamic programming in adaptive sampling space : MATLAB Function  TreatAsAtomicUnit=on
  increase DP path nodes : MATLAB Function  TreatAsAtomicUnit=on
  increase DP path nodes1 : MATLAB Function  TreatAsAtomicUnit=on
  path decision with dynamic planning(dp) : MATLAB Function  TreatAsAtomicUnit=on
  dp_path_s_final : Outport
  dp_path_l_final : Outport  Port=2
  dp_path_dl_final : Outport  Port=3
  dp_path_ddl_final : Outport  Port=4
  dp_path_l_final_average : Outport  Port=5
  wires:
  [plan_start_s] -> path decision with dynamic planning(dp)/3(plan_start_s)
  path decision with dynamic planning(dp)/2(dp_path_s) -> Scope2/1, [dp_path_s_init]
  increase DP path nodes/2(dp_path_l_final) -> [dp_path_l_final_average]
  [static_obs_l_set] -> path decision with dynamic planning(dp)/2(obs_l_set)
  [plan_start_ddl] -> path decision with dynamic planning(dp)/6(plan_start_dll)
  [plan_start_l] -> path decision with dynamic planning(dp)/4(plan_start_l)
  [static_obs_s_set] -> path decision with dynamic planning(dp)/1(obs_s_set)
  [plan_start_dl] -> increase DP path nodes/5(plan_start_dl)
  increase DP path nodes/4(dp_path_ddl_final) -> [dp_path_ddl_final_average]
  increase DP path nodes/1(dp_path_s_final) -> [dp_path_s_final_average]
  increase DP path nodes/3(dp_path_dl_final) -> [dp_path_dl_final_average]
  path decision with dynamic planning(dp)/3(dp_path_l) -> Scope1/1, [dp_path_l_init]
  [plan_start_l] -> increase DP path nodes/4(plan_start_l)
  [plan_start_ddl] -> increase DP path nodes/6(plan_start_ddl)
  [plan_start_dl] -> path decision with dynamic planning(dp)/5(plan_start_dl)
  [plan_start_s] -> increase DP path nodes/3(plan_start_s)
  [dp_path_l_init] -> increase DP path nodes/2(dp_path_l_init)
  [dp_path_s_init] -> increase DP path nodes/1(dp_path_s_init)
  static_obs_s_set/1 -> [static_obs_s_set]
  static_obs_l_set/1 -> [static_obs_l_set]
  plan_start_s/1 -> [plan_start_s]
  plan_start_l/1 -> [plan_start_l]
  plan_start_dl/1 -> [plan_start_dl]
  plan_start_ddl/1 -> [plan_start_ddl]
  [dp_path_s_final] -> dp_path_s_final/1
  [dp_path_l_final] -> dp_path_l_final/1
  [dp_path_dl_final] -> dp_path_dl_final/1
  [dp_path_ddl_final] -> dp_path_ddl_final/1
  [dp_cost_collision] -> path decision with dynamic planning(dp)/7(w_cost_collision)
  [dp_cost_dl] -> path decision with dynamic planning(dp)/8(w_cost_smooth_dl)
  [dp_cost_ddl] -> path decision with dynamic planning(dp)/9(w_cost_smooth_ddl)
  [dp_cost_dddl] -> path decision with dynamic planning(dp)/10(w_cost_smooth_dddl)
  [dp_cost_ref] -> path decision with dynamic planning(dp)/11(w_cost_ref)
  [dp_row] -> path decision with dynamic planning(dp)/12(row)
  [dp_col] -> path decision with dynamic planning(dp)/13(col)
  [dp_sample_s] -> path decision with dynamic planning(dp)/14(sample_s)
  [dp_sample_l] -> path decision with dynamic planning(dp)/15(sample_l)
  dp_cost_dl/1 -> [dp_cost_dl]
  dp_cost_ddl/1 -> [dp_cost_ddl]
  dp_cost_dddl/1 -> [dp_cost_dddl]
  dp_cost_ref/1 -> [dp_cost_ref]
  dp_row/1 -> [dp_row]
  dp_col/1 -> [dp_col]
  dp_sample_l/1 -> [dp_sample_l]
  dp_sample_s/1 -> [dp_sample_s]
  dp_cost_collision/1 -> [dp_cost_collision]
  [static_obs_s_set] -> Adaptive sampling/6(obs_s_set)
  [static_obs_l_set] -> Adaptive sampling/7(obs_l_set)
  [plan_start_s] -> Adaptive sampling/1(plan_start_s)
  [dp_row] -> Adaptive sampling/2(row)
  [dp_col] -> Adaptive sampling/3(col)
  [dp_sample_s] -> Adaptive sampling/4(sample_s)
  [dp_sample_l] -> Adaptive sampling/5(sample_l)
  Constant/1 -> Adaptive sampling/9(coeff_ref)
  Constant1/1 -> Adaptive sampling/10(coeff_obs)
  Constant2/1 -> Adaptive sampling/11(coeff_bound)
  dynamic programming in adaptive sampling space/2(dp_path_s) -> [dp_path_s_init_1]
  [dp_path_s_init_1] -> increase DP path nodes1/1(dp_path_s_init)
  [plan_start_s] -> increase DP path nodes1/3(plan_start_s)
  [plan_start_l] -> increase DP path nodes1/4(plan_start_l)
  [plan_start_ddl] -> increase DP path nodes1/6(plan_start_ddl)
  [dp_path_l_init_1] -> increase DP path nodes1/2(dp_path_l_init)
  increase DP path nodes1/1(dp_path_s_final) -> [dp_path_s_final]
  increase DP path nodes1/4(dp_path_ddl_final) -> [dp_path_ddl_final]
  increase DP path nodes1/3(dp_path_dl_final) -> [dp_path_dl_final]
  increase DP path nodes1/2(dp_path_l_final) -> [dp_path_l_final]
  [plan_start_dl] -> increase DP path nodes1/5(plan_start_dl)
  [static_obs_s_set] -> dynamic programming in adaptive sampling space/2(obs_s_set)
  [static_obs_l_set] -> dynamic programming in adaptive sampling space/3(obs_l_set)
  [plan_start_s] -> dynamic programming in adaptive sampling space/4(plan_start_s)
  [plan_start_l] -> dynamic programming in adaptive sampling space/5(plan_start_l)
  [plan_start_dl] -> dynamic programming in adaptive sampling space/6(plan_start_dl)
  [plan_start_ddl] -> dynamic programming in adaptive sampling space/7(plan_start_dll)
  [dp_cost_collision] -> dynamic programming in adaptive sampling space/8(w_cost_collision)
  [dp_cost_dl] -> dynamic programming in adaptive sampling space/9(w_cost_smooth_dl)
  [dp_cost_ddl] -> dynamic programming in adaptive sampling space/10(w_cost_smooth_ddl)
  [dp_cost_dddl] -> dynamic programming in adaptive sampling space/11(w_cost_smooth_dddl)
  [dp_cost_ref] -> dynamic programming in adaptive sampling space/12(w_cost_ref)
  [dp_sample_s] -> dynamic programming in adaptive sampling space/13(sample_s)
  [dp_sample_l] -> dynamic programming in adaptive sampling space/14(sample_l)
  Adaptive sampling/1(adaptive_sampling_output) -> dynamic programming in adaptive sampling space/1(adaptive_sampling_output)
  dynamic programming in adaptive sampling space/3(dp_path_l) -> [dp_path_l_init_1]
  qp_path_l_in_last_cycle/1 -> [qp_path_l_in_last_cycle]
  [qp_path_l_in_last_cycle] -> Delay/1
  Delay/1 -> Adaptive sampling/8(qp_path_l)
  [dp_path_l_final_average] -> dp_path_l_final_average/1
  dynamic programming in adaptive sampling space/1(time) -> To Workspace/1
  path decision with dynamic planning(dp)/1(time) -> To Workspace1/1
  dynamic programming in adaptive sampling space/4(minimal_cost) -> To Workspace2/1
  path decision with dynamic planning(dp)/4(minimal_cost) -> To Workspace4/1
  Ground_1/1 -> To Workspace3/1

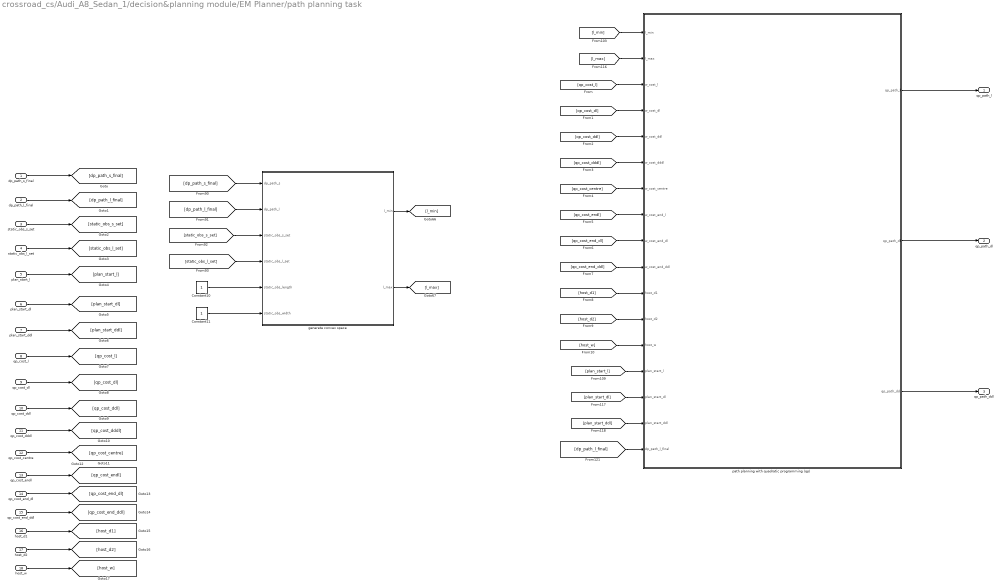
== system crossroad_cs/Audi_A8_Sedan_1/decision&planning module/EM Planner/path planning task ==
  dp_path_s_final : Inport
  dp_path_l_final : Inport  Port=2
  static_obs_s_set : Inport  Port=3
  static_obs_l_set : Inport  Port=4
  plan_start_l : Inport  Port=5
  plan_start_dl : Inport  Port=6
  plan_start_ddl : Inport  Port=7
  qp_cost_l : Inport  Port=8
  qp_cost_dl : Inport  Port=9
  qp_cost_ddl : Inport  Port=10
  qp_cost_dddl : Inport  Port=11
  qp_cost_centre : Inport  Port=12
  qp_cost_endl : Inport  Port=13
  qp_cost_end_dl : Inport  Port=14
  qp_cost_end_ddl : Inport  Port=15
  host_d1 : Inport  Port=16
  host_d2 : Inport  Port=17
  host_w : Inport  Port=18
  Constant10 : Constant
  Constant11 : Constant
  generate convex space : MATLAB Function  TreatAsAtomicUnit=on
  path planning with quadratic programming (qp) : MATLAB Function  TreatAsAtomicUnit=on
  qp_path_l : Outport
  qp_path_dl : Outport  Port=2
  qp_path_ddl : Outport  Port=3
  wires:
  generate convex space/2(l_max) -> [l_max]
  Constant11/1 -> generate convex space/6(static_obs_width)
  Constant10/1 -> generate convex space/5(static_obs_length)
  [static_obs_l_set] -> generate convex space/4(static_obs_l_set)
  [dp_path_l_final] -> path planning with quadratic programming (qp)/17(dp_path_l_final)
  [dp_path_s_final] -> generate convex space/1(dp_path_s)
  path planning with quadratic programming (qp)/1(qp_path_l) -> qp_path_l/1
  [plan_start_l] -> path planning with quadratic programming (qp)/14(plan_start_l)
  generate convex space/1(l_min) -> [l_min]
  [static_obs_s_set] -> generate convex space/3(static_obs_s_set)
  [dp_path_l_final] -> generate convex space/2(dp_path_l)
  [plan_start_dl] -> path planning with quadratic programming (qp)/15(plan_start_dl)
  [l_max] -> path planning with quadratic programming (qp)/2(l_max)
  [l_min] -> path planning with quadratic programming (qp)/1(l_min)
  [plan_start_ddl] -> path planning with quadratic programming (qp)/16(plan_start_ddl)
  path planning with quadratic programming (qp)/3(qp_path_ddl) -> qp_path_ddl/1
  path planning with quadratic programming (qp)/2(qp_path_dl) -> qp_path_dl/1
  dp_path_s_final/1 -> [dp_path_s_final]
  dp_path_l_final/1 -> [dp_path_l_final]
  static_obs_s_set/1 -> [static_obs_s_set]
  static_obs_l_set/1 -> [static_obs_l_set]
  plan_start_l/1 -> [plan_start_l]
  plan_start_dl/1 -> [plan_start_dl]
  plan_start_ddl/1 -> [plan_start_ddl]
  [qp_cost_l] -> path planning with quadratic programming (qp)/3(w_cost_l)
  [qp_cost_dl] -> path planning with quadratic programming (qp)/4(w_cost_dl)
  [qp_cost_ddl] -> path planning with quadratic programming (qp)/5(w_cost_ddl)
  [qp_cost_dddl] -> path planning with quadratic programming (qp)/6(w_cost_dddl)
  [qp_cost_centre] -> path planning with quadratic programming (qp)/7(w_cost_centre)
  [qp_cost_endl] -> path planning with quadratic programming (qp)/8(w_cost_end_l)
  [qp_cost_end_dl] -> path planning with quadratic programming (qp)/9(w_cost_end_dl)
  [qp_cost_end_ddl] -> path planning with quadratic programming (qp)/10(w_cost_end_ddl)
  [host_d1] -> path planning with quadratic programming (qp)/11(host_d1)
  [host_d2] -> path planning with quadratic programming (qp)/12(host_d2)
  [host_w] -> path planning with quadratic programming (qp)/13(host_w)
  qp_cost_l/1 -> [qp_cost_l]
  qp_cost_dl/1 -> [qp_cost_dl]
  qp_cost_ddl/1 -> [qp_cost_ddl]
  qp_cost_dddl/1 -> [qp_cost_dddl]
  qp_cost_centre/1 -> [qp_cost_centre]
  qp_cost_endl/1 -> [qp_cost_endl]
  qp_cost_end_dl/1 -> [qp_cost_end_dl]
  qp_cost_end_ddl/1 -> [qp_cost_end_ddl]
  host_d1/1 -> [host_d1]
  host_d2/1 -> [host_d2]
  host_w/1 -> [host_w]

== system crossroad_cs/Box_1/SELF_Demux/compas converter/cart2compas ==
  Angle [deg] : Inport
  Constant : Constant  Value=90
  Constant1 : Constant  Value=360
  Gain : Gain  Gain=1/360
  Gain1 : Gain  Gain=360
  Gain2 : Gain  Gain=-1
  Rounding Function : Rounding
  Sum : Sum  Inputs=|-+
  Sum1 : Sum  Inputs=-+|
  Sum2 : Sum  Inputs=++|
  heading [deg] : Outport
  wires:
  Gain/1 -> Rounding Function/1
  Rounding Function/1 -> Gain1/1
  Gain1/1 -> Sum/1
  Angle [deg]/1 -> Sum1/2
  Sum/1 -> Gain2/1
  Sum1/1 -> Gain/1, Sum/2
  Constant/1 -> Sum1/1
  Gain2/1 -> Sum2/2
  Constant1/1 -> Sum2/1
  Sum2/1 -> heading [deg]/1

== system crossroad_cs/Box_2/SELF_Demux/compas converter/cart2compas ==
  Angle [deg] : Inport
  Constant : Constant  Value=90
  Constant1 : Constant  Value=360
  Gain : Gain  Gain=1/360
  Gain1 : Gain  Gain=360
  Gain2 : Gain  Gain=-1
  Rounding Function : Rounding
  Sum : Sum  Inputs=|-+
  Sum1 : Sum  Inputs=-+|
  Sum2 : Sum  Inputs=++|
  heading [deg] : Outport
  wires:
  Gain/1 -> Rounding Function/1
  Rounding Function/1 -> Gain1/1
  Gain1/1 -> Sum/1
  Angle [deg]/1 -> Sum1/2
  Sum/1 -> Gain2/1
  Sum1/1 -> Gain/1, Sum/2
  Constant/1 -> Sum1/1
  Gain2/1 -> Sum2/2
  Constant1/1 -> Sum2/1
  Sum2/1 -> heading [deg]/1

== system crossroad_cs/Box_3/SELF_Demux/compas converter/cart2compas ==
  Angle [deg] : Inport
  Constant : Constant  Value=90
  Constant1 : Constant  Value=360
  Gain : Gain  Gain=1/360
  Gain1 : Gain  Gain=360
  Gain2 : Gain  Gain=-1
  Rounding Function : Rounding
  Sum : Sum  Inputs=|-+
  Sum1 : Sum  Inputs=-+|
  Sum2 : Sum  Inputs=++|
  heading [deg] : Outport
  wires:
  Gain/1 -> Rounding Function/1
  Rounding Function/1 -> Gain1/1
  Gain1/1 -> Sum/1
  Angle [deg]/1 -> Sum1/2
  Sum/1 -> Gain2/1
  Sum1/1 -> Gain/1, Sum/2
  Constant/1 -> Sum1/1
  Gain2/1 -> Sum2/2
  Constant1/1 -> Sum2/1
  Sum2/1 -> heading [deg]/1

== system crossroad_cs/Box_4/SELF_Demux/compas converter/cart2compas ==
  Angle [deg] : Inport
  Constant : Constant  Value=90
  Constant1 : Constant  Value=360
  Gain : Gain  Gain=1/360
  Gain1 : Gain  Gain=360
  Gain2 : Gain  Gain=-1
  Rounding Function : Rounding
  Sum : Sum  Inputs=|-+
  Sum1 : Sum  Inputs=-+|
  Sum2 : Sum  Inputs=++|
  heading [deg] : Outport
  wires:
  Gain/1 -> Rounding Function/1
  Rounding Function/1 -> Gain1/1
  Gain1/1 -> Sum/1
  Angle [deg]/1 -> Sum1/2
  Sum/1 -> Gain2/1
  Sum1/1 -> Gain/1, Sum/2
  Constant/1 -> Sum1/1
  Gain2/1 -> Sum2/2
  Constant1/1 -> Sum2/1
  Sum2/1 -> heading [deg]/1

== system crossroad_cs/Audi_A8_Sedan_1/control module1/control main/longitudinal control double PID/discrete pid ==
  err : Inport
  kp : Inport  Port=2
  ki : Inport  Port=3
  kd : Inport  Port=4
  Add2 : Sum  Inputs=+++
  Add3 : Sum
  Add4 : Sum  Inputs=+-
  Delay3 : Delay  DelayLength=1
  Delay4 : Delay  DelayLength=1
  Divide : Product  Inputs=**
  Divide1 : Product  Inputs=**
  Divide2 : Product  Inputs=**
  Gain : Gain  Gain=0.01
  pid_out : Outport
  wires:
  [KD_PID_distance] -> Divide2/2
  err/1 -> Delay4/1, Divide/2, Add3/1, Add4/1
  Divide/1 -> Add2/1
  Divide2/1 -> Add2/3
  Add3/1 -> Gain/1, Divide1/1
  Delay4/1 -> Add4/2
  [KP_PID_distance] -> Divide/1
  Divide1/1 -> Add2/2
  Delay3/1 -> Add3/2
  [KI_PID_distance] -> Divide1/2
  Add4/1 -> Divide2/1
  Add2/1 -> pid_out/1
  kp/1 -> [KP_PID_distance]
  ki/1 -> [KI_PID_distance]
  kd/1 -> [KD_PID_distance]
  Gain/1 -> Delay3/1
